simulink model "Control_Jetson_10ms_21b 1"  (R2021b)
settings: Solver=ode4  StartTime=0.0  StopTime=10  FixedStep=0.01  MaxStep=0  RelTol=1e-5  AbsTol=1e-3
InitFcn:
  | % Carrega parâmetros gerais (Massa, Ganhos PID, Geometria)
  | run('Parameters.m');
  | 
  | % Carrega as Tabelas (Lookup Tables)
  | run('curva_steering.m');
  | run('curva_tq_motor.m');
  | Ts = 0.001;
  | % (Opcional) Mensagem no Command Window para confirmar que rodou
  | disp('--- Parâmetros e Curvas Carregados com Sucesso ---');
model workspace (MAT data in the model file):
  A = 1.22
  Ack = 1
  Cd = 1.1
  Cl = -2
  Cs = [19075.58 25992.8 31792.64 35898.02 39044.37]
  Fz0x = -811.9083
  Fz0y = -210.9467
  Fz_cs = [222.41 444.82 667.23 889.64 1112.05]
  IAY = 0
  IAx = 0
  IAy = 0
  Im = 0.00033
  It = 0.0094
  Iw = 0.1578
  Iw_ = 0.7
  Iz_car = 150
  K_50_understeer = 0.005184
  K_Stability = 1
  K_oversteer = -0.001
  Kappa_F = 0
  Kappa_R = 0
  Km_FM = 110000
  Km_Fm = 110000
  Km_RM = 120000
  Km_Rm = 120000
  KphiARB_F = 0
  KphiARB_R = 11000
  KphiF = 1068.14
  KphiR = 1637.12
  Kphim_F = 137500
  Kphim_R = 48600
  L = 1.53
  M = 300
  Mgt = 11.72
  Mz_maxF = [0 66.3 132.6 198.9 265.2 330.23 396.52 462.83 529.112 595.42 661.73 728.03 794.33 860.62 926.92 993.23 1058.25 1124.55 1190.85 1257.15 1323.45 1389.75 1456.05 1522.35 1588.65 1654.95]
  Mz_minF = [0 -66.3 -132.6 -198.9 -265.2 -330.23 -396.52 -462.83 -529.112 -595.42 -661.73 -728.03 -794.33 -860.62 -926.92 -993.23 -1058.25 -1124.55 -1190.85 -1257.15 -1323.45 -1389.75 -1456.05 -1522.35 -1588.65 -1654.95]
  P = 68.9476
  P0 = 55.4852
  R = 0.2032
  Rcurva = 20
  Re = 0.2
  SR = 3
  TV_On = 1
  Ts = 0.01
  W = 2940
  Wf = 661.5
  Wr = 808.5
  Ws = 2324
  YLL = 1.11022302463e-16
  cx1 = 1.3668
  cy1 = 1.839
  dpi = 0.242630467224
  dx1 = 2.1568
  dx2 = -0.065814
  dx3 = 0.0011254
  dy1 = 2.453
  dy2 = -0.11197
  dy3 = 10.2899
  ex1 = -0.19815
  ex2 = -0.62529
  ex3 = 1.3396
  ex4 = 0.0029464
  ey1 = 0.96085
  ey2 = -0.28662
  ey3 = 0.14389
  ey4 = 4.9274
  ey5 = -70.7165
  g = 9.8
  hcg = 0.28495
  hcgs = 0.202
  hrc_f = 0.065
  hrc_r = 0.094
  hs_f = 0.245
  hs_r = 0.21
  hx1 = -0.003859
  hx2 = -0.000374
  hy1 = -0.000403
  hy2 = -0.000261
  kx1 = -36.9039
  kx2 = 22.3857
  kx3 = 0.61844
  ky1 = -83.2526
  ky2 = -5.565
  ky3 = 0.88491
  ky4 = 2.9994
  ky5 = -99.9393
  ky6 = -3.4705
  ky7 = -0.91452
  lf = 0.8415
  lr = 0.6885
  mass_FL = 67.5
  mass_FR = 67.5
  mass_RL = 82.5
  mass_RR = 82.5
  mi = 2
  ms = 240
  pedal = [0 1 2 3 4 5 6 7 8 9 10 11 12 13 14 15 16 17 18 19 20 21 22 23 24 25]
  pty1 = 0.005744
  pty2 = 19.1334
  px1 = -0.039964
  px2 = -0.15015
  px3 = -0.32528
  px4 = -0.063273
  py1 = 0.38578
  py2 = 1.2048
  py3 = -0.14544
  py4 = 0.092886
  py5 = -0.82901
  r = 9
  rhoar = 1.22
  s_f = 1
  s_r = 0.9
  tf = 1.2
  tr = 1.18
  vx1 = -0.11922
  vx2 = 0.002205
  vy1 = 0.032907
  vy2 = 0.018068
  vy3 = -1.0429
  vy4 = 0.53712
  x_fl = 0.8415
  x_fr = 0.8415
  x_rl = 0.6885
  x_rr = 0.6885
  xs_f = 0.89
  xs_r = 0.638
  y_fl = 0.6
  y_fr = 0.6
  y_rl = 0.59
  y_rr = 0.59
undefined symbols (not defined in the file or in its folder): Gr, K_t, K_variavel, Ki_data, Kp_data, magnitude, rpm, torque, Vx, Vx_axis
libraries: simulink x10, fuzblock x4
(part 1 of 2)
settings Model: SimulationMode=accelerator  NumberOfSteps=275  Creator=lucas  LastModifiedBy=Aline
settings SolverCC: ZeroCrossAlgorithm=Adaptive
settings DebuggingCC: SignalInfNanChecking=error  IgnoredZcDiagnostic=none  UnconnectedInputMsg=none  UnconnectedOutputMsg=none  UnconnectedLineMsg=none
settings ModelReferenceCC: EnableRefExpFcnMdlSchedulingChecks=off
settings RTWCC: GPUComputeCapability=5.0  DLArmComputeVersion=20.02.1

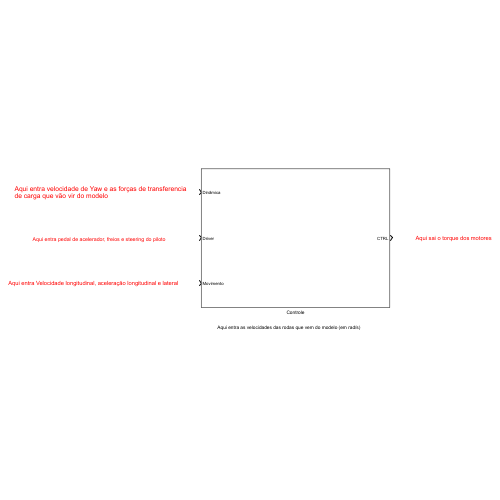
[thumbnail: Simulink's stored preview of the top-level diagram]
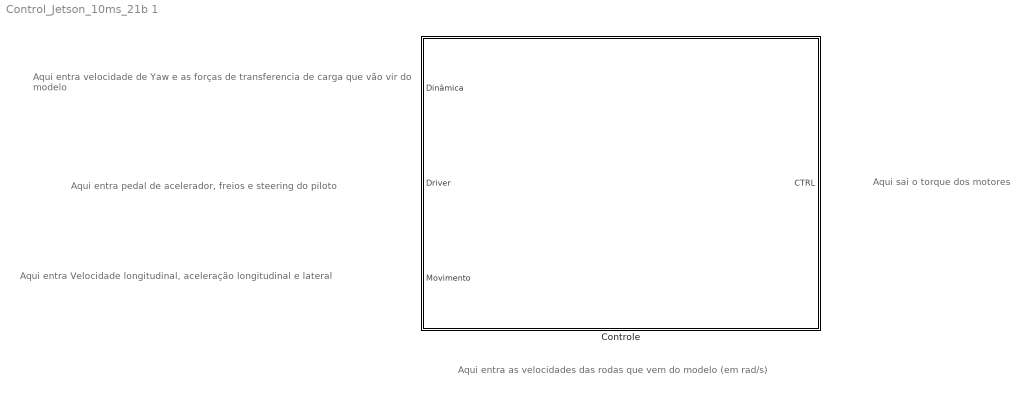
== system Control_Jetson_10ms_21b 1 ==
  note: Aqui sai o torque dos motores
  note: Aqui entra as velocidades das rodas que vem do modelo (em rad/s)
  note: Aqui entra Velocidade longitudinal, aceleração longitudinal e lateral
  note: Aqui entra pedal de acelerador, freios e steering do piloto
  note: Aqui entra velocidade de Yaw e as forças de transferencia
      | de carga que vão vir do modelo
  Controle : Subsystem

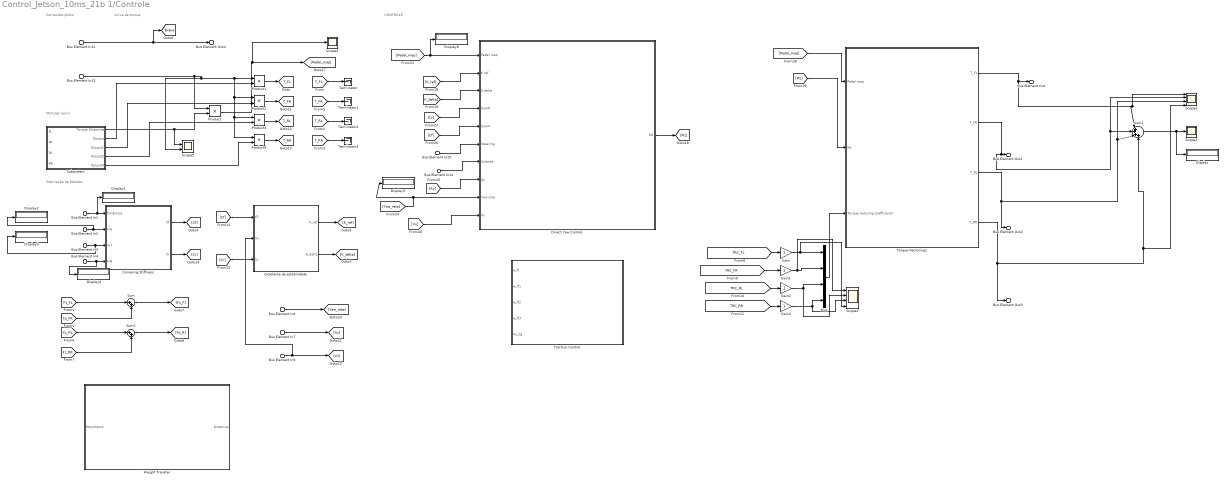
== system Control_Jetson_10ms_21b 1/Controle ==
  note: CONTROLE
  note: Estimação de Estados
  note: Motores
      |  (rpm)
  note: Comandos piloto
  note: curva de torque
  Bus Element In1 : Inport  PortName=Dinâmica  Element=Fz_FL
  Bus Element In2 : Inport  PortName=Dinâmica  Element=Fz_FR
  Bus Element In3 : Inport  PortName=Dinâmica  Element=Fz_RL
  Bus Element In4 : Inport  PortName=Dinâmica  Element=Fz_RR
  Bus Element In6 : Inport  PortName=Dinâmica  Element=Yaw.v_yaw
  Bus Element In12 : Inport  Port=2  PortName=Driver  Element=BrakeCmd
  Bus Element In13 : Inport  Port=2  PortName=Driver  Element=AccCmd
  Bus Element In14 : Inport  Port=2  PortName=Driver  Element=volante
  Bus Element In15 : Inport  Port=2  PortName=Driver  Element=steering_inner
  Bus Element In5 : Inport  Port=3  PortName=Movimento  Element=Vx_cg
  Bus Element In7 : Inport  Port=3  PortName=Movimento  Element=Ay_cg
  Cornering Stiffness : Subsystem
  Direct Yaw Control : Subsystem
  Display{,1..6} (7 alike) : Display
  Gain{,1..3} (4 alike) : Gain
  Gradiente de estabilidade : Subsystem
  Mux : Mux
  Product{,1..4} (5 alike) : Product
  Scope1 : Scope
  Scope2 : Scope  NumInputPorts=4
  Scope3 : Scope  NumInputPorts=4
  Scope4 : Scope
  Scope5 : Scope  NumInputPorts=2
  Subsystem : Subsystem
  Sum : Sum  Inputs=|++
  Sum1 : Sum  Inputs=|++
  Sum2 : Sum  Inputs=|++++
  Terminator{,1..3} (4 alike) : Terminator
  Torque Vectoring1 : Subsystem
  Traction Control : Subsystem
  "Weight Transfer " : Subsystem
  Bus Element Out4 : Outport  PortName=CTRL  Element=BrakeCmd
  Bus Element Out : Outport  VectorParamsAs1DForOutWhenUnconnected=off  PortName=CTRL  Element=T_FL
  Bus Element Out1 : Outport  VectorParamsAs1DForOutWhenUnconnected=off  PortName=CTRL  Element=T_FR
  Bus Element Out2 : Outport  VectorParamsAs1DForOutWhenUnconnected=off  PortName=CTRL  Element=T_RL
  Bus Element Out3 : Outport  VectorParamsAs1DForOutWhenUnconnected=off  PortName=CTRL  Element=T_RR
  tag scope: Brake=global, T_FL=global, T_FR=global, T_RL=global, T_RR=global
  wires:
  Gradiente de estabilidade/2(K_delta) -> [K_delta]
  Bus Element In13/1 -> Scope5/2, Product4/1, Product3/1, Product2/1, Product1/1, Product/1
  Bus Element In12/1 -> [Brake], Bus Element Out4/1
  Cornering Stiffness/1(Cf) -> [Cf]
  Cornering Stiffness/2(Cr) -> [Cr]
  Bus Element In3/1 -> Display3/1, Cornering Stiffness/3(In7)
  Bus Element In1/1 -> Display1/1, Cornering Stiffness/1(Dinâmica)
  Bus Element In4/1 -> Display4/1, Cornering Stiffness/4(In8)
  Bus Element In2/1 -> Display2/1, Cornering Stiffness/2(In6)
  [Cr] -> Gradiente de estabilidade/3(Cr)
  [Cf] -> Gradiente de estabilidade/1(Cf)
  Gradiente de estabilidade/1(K_ref) -> [K_ref]
  Direct Yaw Control/1(Mz) -> [Mz]
  Bus Element In14/1 -> Direct Yaw Control/7(Volante)
  Bus Element In15/1 -> Direct Yaw Control/6(Steering)
  [Mz] -> Torque Vectoring1/2(Mz)
  Sum/1 -> [Fz_F]
  Sum1/1 -> [Fz_R]
  Bus Element In5/1 -> Gradiente de estabilidade/2(Vx), [Vx]
  Bus Element In7/1 -> [Ay]
  Bus Element In6/1 -> [Yaw_rate]
  [T_FL] -> Terminator/1
  [T_FR] -> Terminator1/1
  [T_RL] -> Terminator2/1
  [T_RR] -> Terminator3/1
  Sum2/1 -> Display/1, Scope1/1
  Mux/1 -> Torque Vectoring1/3(Torque reducing coefficients)
  Product/1 -> [Pedal_map], Scope4/1
  Subsystem/1(Torque Disponivel) -> Product/2, Scope5/1
  Product1/1 -> [T_FL]
  Product2/1 -> [T_FR]
  Product3/1 -> [T_RL]
  Product4/1 -> [T_RR]
  Subsystem/5(Output3) -> Product4/2
  Subsystem/4(Output2) -> Product3/2
  Subsystem/3(Output1) -> Product2/2
  Subsystem/2(Output) -> Product1/2
  ? -> Subsystem/3(RL)
  ? -> Subsystem/4(RR)
  ? -> Subsystem/2(FR)
  ? -> Subsystem/1(FL)
  Torque Vectoring1/2(T_FR) -> Scope3/2, Sum2/2, Bus Element Out1/1
  Torque Vectoring1/3(T_RL) -> Bus Element Out2/1, Scope3/3, Sum2/3
  Torque Vectoring1/1(T_FL) -> Sum2/1, Scope3/1, Bus Element Out/1
  Torque Vectoring1/4(T_RR) -> Bus Element Out3/1, Scope3/4, Sum2/4
  [TRC_FL] -> Gain/1
  [TRC_FR] -> Gain1/1
  Gain/1 -> Scope2/4, Mux/1
  Gain1/1 -> Scope2/1, Mux/2
  [TRC_RL] -> Gain2/1
  [TRC_RR] -> Gain3/1
  [Pedal_map] -> Direct Yaw Control/1(Pedal map), Display6/1
  [K_ref] -> Direct Yaw Control/2(K ref)
  [K_delta] -> Direct Yaw Control/3(K delta)
  [Cr] -> Direct Yaw Control/4(CornR)
  [Cf] -> Direct Yaw Control/5(CornF)
  [Ay] -> Direct Yaw Control/8(Ay)
  [Vx] -> Direct Yaw Control/10(Vx)
  [Pedal_map] -> Torque Vectoring1/1(Pedal map)
  Gain2/1 -> Mux/3, Scope2/2
  Gain3/1 -> Mux/4, Scope2/3
  [Yaw_rate] -> Direct Yaw Control/9(Yaw rate), Display5/1
  [Fz_FR] -> Sum/2
  [Fz_FL] -> Sum/1
  [Fz_RR] -> Sum1/2
  [Fz_RL] -> Sum1/1

== system Control_Jetson_10ms_21b 1/Controle/Cornering Stiffness ==
  Dinâmica : Inport
  In6 : Inport  Port=2
  In7 : Inport  Port=3
  In8 : Inport  Port=4
  1-D Lookup Table{,1..3} (4 alike) : Lookup_n-D  NumberOfTableDimensions=1  BreakpointsForDimension1=Fz_cs  Table=Cs  InternalRulePriority=Speed  RndMeth=Simplest  InputSameDT=on
  Sum : Sum  Inputs=|++
  Sum1 : Sum  Inputs=|++
  Cf : Outport
  Cr : Outport  Port=2
  wires:
  1-D Lookup Table1/1 -> Sum1/2
  In7/1 -> 1-D Lookup Table2/1
  Sum/1 -> Cr/1
  Sum1/1 -> Cf/1
  Dinâmica/1 -> 1-D Lookup Table/1
  In6/1 -> 1-D Lookup Table1/1
  1-D Lookup Table3/1 -> Sum/2
  1-D Lookup Table/1 -> Sum1/1
  1-D Lookup Table2/1 -> Sum/1
  In8/1 -> 1-D Lookup Table3/1

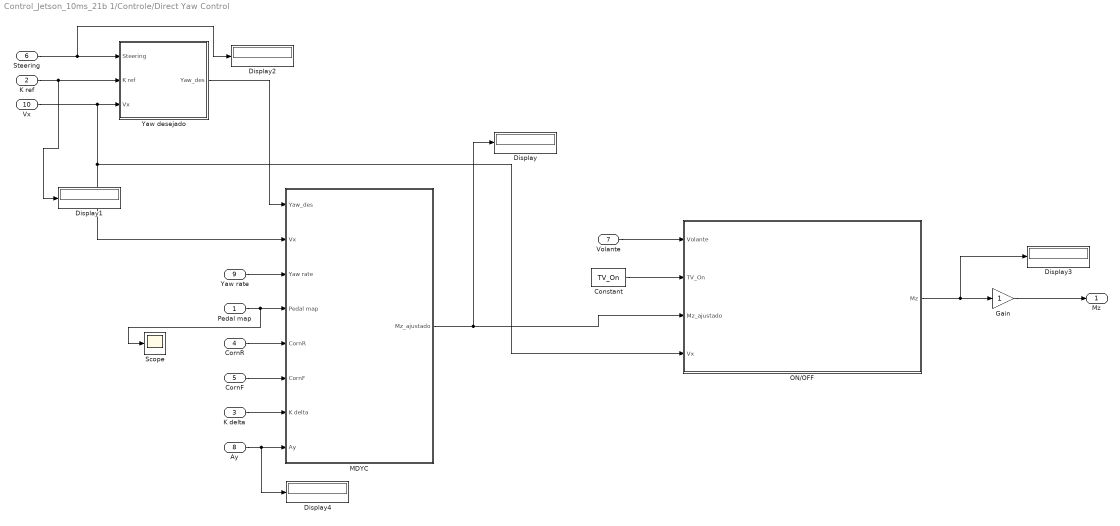
== system Control_Jetson_10ms_21b 1/Controle/Direct Yaw Control ==
  Pedal map : Inport
  K ref : Inport  Port=2
  K delta : Inport  Port=3
  CornR : Inport  Port=4
  CornF : Inport  Port=5
  Steering : Inport  Port=6
  Volante : Inport  Port=7
  Ay : Inport  Port=8
  Yaw rate : Inport  Port=9
  Vx : Inport  Port=10
  Constant : Constant  Value=TV_On
  Display{,1..4} (5 alike) : Display
  Gain : Gain
  MDYC : Subsystem
  ON/OFF : Subsystem
  Scope : Scope
  Yaw desejado : Subsystem
  Mz : Outport
  wires:
  Steering/1 -> Display2/1, Yaw desejado/1(Steering)
  K ref/1 -> Display1/1, Yaw desejado/2(K ref)
  Vx/1 -> MDYC/2(Vx), ON/OFF/4(Vx), Yaw desejado/3(Vx)
  Yaw desejado/1(Yaw_des) -> MDYC/1(Yaw_des)
  Yaw rate/1 -> MDYC/3(Yaw rate)
  Pedal map/1 -> Scope/1, MDYC/4(Pedal map)
  CornR/1 -> MDYC/5(CornR)
  CornF/1 -> MDYC/6(CornF)
  K delta/1 -> MDYC/7(K delta)
  Ay/1 -> Display4/1, MDYC/8(Ay)
  Volante/1 -> ON/OFF/1(Volante)
  Constant/1 -> ON/OFF/2(TV_On)
  MDYC/1(Mz_ajustado) -> Display/1, ON/OFF/3(Mz_ajustado)
  ON/OFF/1(Mz) -> Display3/1, Gain/1
  Gain/1 -> Mz/1

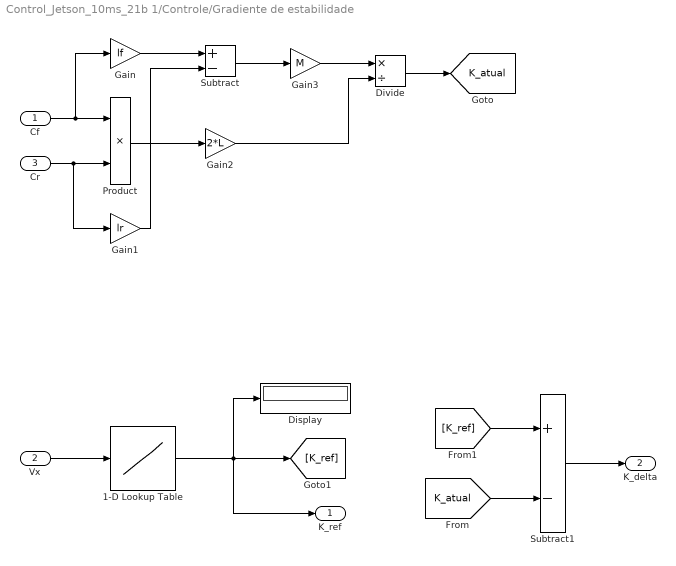
== system Control_Jetson_10ms_21b 1/Controle/Gradiente de estabilidade ==
  Cf : Inport
  Vx : Inport  Port=2
  Cr : Inport  Port=3
  1-D Lookup Table : Lookup_n-D  NumberOfTableDimensions=1  BreakpointsForDimension1=Vx  Table=K_variavel  InternalRulePriority=Speed  RndMeth=Simplest  InputSameDT=on
  Display : Display
  Divide : Product  Inputs=*/
  Gain : Gain  Gain=lf
  Gain1 : Gain  Gain=lr
  Gain2 : Gain  Gain=2*L
  Gain3 : Gain  Gain=M
  Product : Product
  Subtract : Sum  Inputs=+-
  Subtract1 : Sum  Inputs=+-
  K_ref : Outport
  K_delta : Outport  Port=2
  tag scope: K_atual=global
  wires:
  Cr/1 -> Product/2, Gain1/1
  [K_ref] -> Subtract1/1
  Product/1 -> Gain2/1
  Divide/1 -> [K_atual]
  Subtract1/1 -> K_delta/1
  Gain2/1 -> Divide/2
  [K_atual] -> Subtract1/2
  Gain3/1 -> Divide/1
  Cf/1 -> Gain/1, Product/1
  Gain1/1 -> Subtract/2
  Gain/1 -> Subtract/1
  Subtract/1 -> Gain3/1
  Vx/1 -> 1-D Lookup Table/1
  1-D Lookup Table/1 -> Display/1, K_ref/1, [K_ref]

== system Control_Jetson_10ms_21b 1/Controle/Subsystem ==
  Bus Element In1 : Inport  PortName=FL
  Bus Element In2 : Inport  Port=2  PortName=FR
  Bus Element In3 : Inport  Port=3  PortName=RL
  Bus Element In4 : Inport  Port=4  PortName=RR
  1-D Lookup Table{,1..3} (4 alike) : Lookup_n-D  NumberOfTableDimensions=1  BreakpointsForDimension1=rpm  Table=torque  InternalRulePriority=Speed  RndMeth=Simplest  InputSameDT=on
  Sum : Sum  Inputs=|++++
  Torque Disponivel : Outport
  Output : Outport  Port=2
  Output1 : Outport  Port=3
  Output2 : Outport  Port=4
  Output3 : Outport  Port=5
  wires:
  1-D Lookup Table/1 -> Output/1, Output1/1, Sum/1
  1-D Lookup Table1/1 -> Sum/2
  1-D Lookup Table2/1 -> Output2/1, Sum/3
  1-D Lookup Table3/1 -> Output3/1, Sum/4
  Sum/1 -> Torque Disponivel/1
  Bus Element In1/1 -> 1-D Lookup Table/1
  Bus Element In2/1 -> 1-D Lookup Table1/1
  Bus Element In3/1 -> 1-D Lookup Table2/1
  Bus Element In4/1 -> 1-D Lookup Table3/1

== system Control_Jetson_10ms_21b 1/Controle/Torque Vectoring1 ==
  note: rever isso daqui
  Pedal map : Inport
  Mz : Inport  Port=2
  Torque reducing coefficients : Inport  Port=3
  Display : Display
  Display1 : Display
  Distribuição Lateral2 : Subsystem
  Distribuição longitudinal : Subsystem
  Redução TC1 : Subsystem
  Scope : Scope  NumInputPorts=4
  Scope1 : Scope  NumInputPorts=2
  Subsystem : Subsystem
  T_FL : Outport
  T_FR : Outport  Port=2
  T_RL : Outport  Port=3
  T_RR : Outport  Port=4
  tag scope: Tq_F=global, Tq_R=global
  wires:
  Redução TC1/3(T_RLreduzido) -> Scope/3, T_RL/1  "RL"
  Torque reducing coefficients/1 -> Redução TC1/1(Torque reducing coefficients)
  Subsystem/2("Tq_R ") -> Distribuição Lateral2/4("Tq_R "), [Tq_R]
  Mz/1 -> Subsystem/1(MzT)
  Redução TC1/2(T_FRreduzido) -> Scope/2, T_FR/1  "FR"
  Redução TC1/1(T_FLreduzido) -> Scope1/2, Scope/1, T_FL/1  "FL"
  Subsystem/1(Tq_F) -> Distribuição Lateral2/3(Tq_F), [Tq_F]
  Redução TC1/4(T_RRreduzido) -> Scope/4, T_RR/1  "RR"
  Distribuição longitudinal/1(Dianteiro) -> Distribuição Lateral2/1(Dianteiro)
  Distribuição longitudinal/2(Traseiro) -> Distribuição Lateral2/2(Traseiro)
  Pedal map/1 -> Distribuição longitudinal/1(In1)
  Distribuição Lateral2/1(TFL_lat) -> Redução TC1/2(TFL)
  Distribuição Lateral2/2(TFR_lat) -> Redução TC1/3(TFR)
  Distribuição Lateral2/3(TRL_lat) -> Redução TC1/4(TRL)
  Distribuição Lateral2/4(TRR_lat) -> Redução TC1/5(TRR)

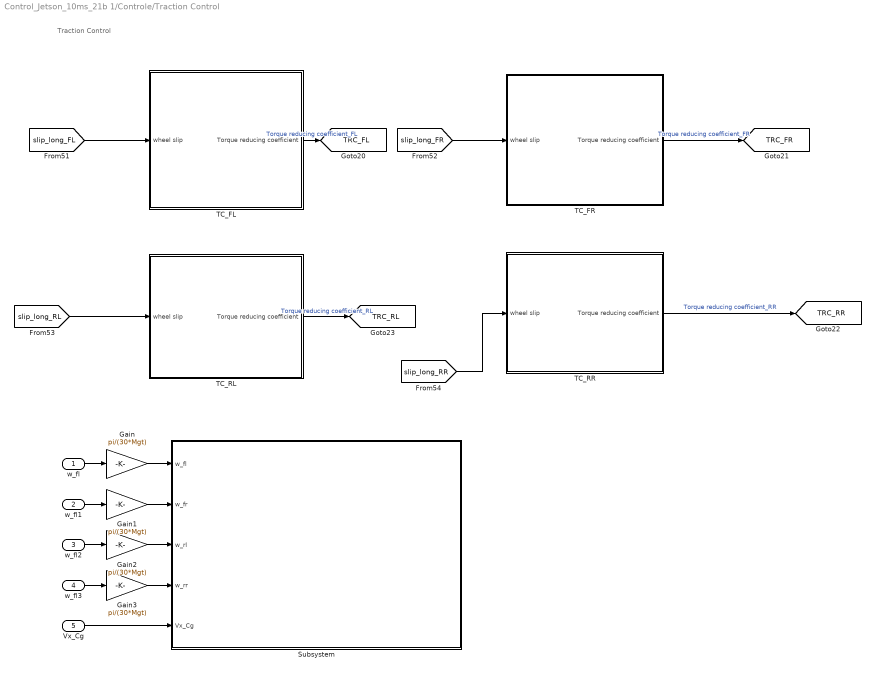
== system Control_Jetson_10ms_21b 1/Controle/Traction Control ==
  note: Traction Control
  w_fl : Inport
  w_fl1 : Inport  Port=2
  w_fl2 : Inport  Port=3
  w_fl3 : Inport  Port=4
  Vx_Cg : Inport  Port=5
  Gain{,1..3} (4 alike) : Gain  Gain=pi/(30*Mgt)
  Subsystem : Subsystem
  TC_FL : Subsystem
  TC_FR : Subsystem
  TC_RL : Subsystem
  TC_RR : Subsystem
  tag scope: TRC_FL=global, TRC_FR=global, TRC_RL=global, TRC_RR=global
  wires:
  TC_FR/1(Torque reducing coefficient) -> [TRC_FR]  "Torque reducing coefficient_FR"
  TC_RL/1(Torque reducing coefficient) -> [TRC_RL]  "Torque reducing coefficient_RL"
  TC_FL/1(Torque reducing coefficient) -> [TRC_FL]  "Torque reducing coefficient_FL"
  [slip_long_FL] -> TC_FL/1(wheel slip)
  [slip_long_RL] -> TC_RL/1(wheel slip)
  [slip_long_RR] -> TC_RR/1(wheel slip)
  [slip_long_FR] -> TC_FR/1(wheel slip)
  TC_RR/1(Torque reducing coefficient) -> [TRC_RR]  "Torque reducing coefficient_RR"
  w_fl/1 -> Gain/1
  w_fl1/1 -> Gain1/1
  w_fl2/1 -> Gain2/1
  w_fl3/1 -> Gain3/1
  Gain/1 -> Subsystem/1(w_fl)
  Gain1/1 -> Subsystem/2(w_fr)
  Gain2/1 -> Subsystem/3(w_rl)
  Gain3/1 -> Subsystem/4(w_rr)
  Vx_Cg/1 -> Subsystem/5(Vx_Cg)

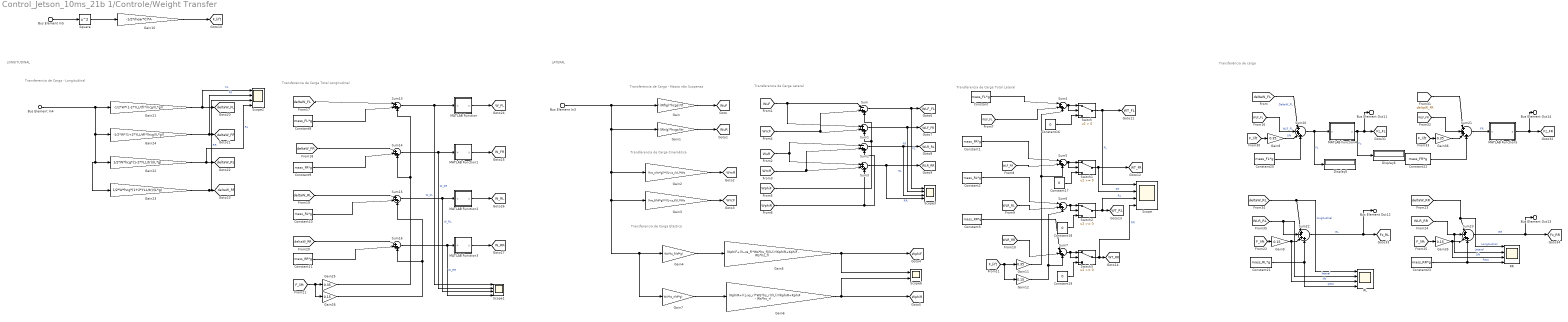
== system Control_Jetson_10ms_21b 1/Controle/Weight Transfer  ==
  note: Transferencia de Carga Lateral
  note: LATERAL
  note: Transferencia de Carga Cinemática
  note: Transferência de carga
  note: Transferencia de Carga - Massa não Suspensa
  note: Transferencia de Carga Total Lateral
  note: LONGITUDINAL
  note: Transferencia de Carga - Longitudinal
  note: Transferencia de Carga Total Longitudinal
  note: Transferencia de Carga Elástica
  Bus Element In3 : Inport  PortName=Movimento  Element=Ay_cg
  Bus Element In4 : Inport  PortName=Movimento  Element=Ax_cg
  Bus Element In5 : Inport  PortName=Movimento  Element=Vx_cg
  Constant : Constant  Value=mass_FL*g
  Constant1 : Constant  Value=mass_FR*g
  Constant10 : Constant  Value=mass_RL*g
  Constant11 : Constant  Value=mass_RR*g
  Constant{16..19} (4 alike) : Constant  Value=0
  Constant2 : Constant  Value=mass_RL*g
  Constant20 : Constant  Value=mass_FL*g
  Constant21 : Constant  Value=mass_RL*g
  Constant22 : Constant  Value=mass_FR*g
  Constant23 : Constant  Value=mass_RR*g
  Constant3 : Constant  Value=mass_RR*g
  Constant8 : Constant  Value=mass_FL*g
  Constant9 : Constant  Value=mass_FR*g
  Display5 : Display
  Display6 : Display
  Gain : Gain  Gain=((Wf/g)*hcgs)/tf
  Gain1 : Gain  Gain=((Wr/g)*hcgs)/tr
  Gain10 : Gain  Gain=-1/2*rhoar*Cl*A
  Gain{8,11,25,36} (4 alike) : Gain  Gain=0.35
  Gain{9,12,26,35} (4 alike) : Gain  Gain=0.15
  Gain2 : Gain  Gain=(hrc_r/(tr*g))*((L-xs_r)/L)*Ws
  Gain21 : Gain  Gain=-1/2*W*(1-2*YLL/tf)*(hcg/(L*g))
  Gain22 : Gain  Gain=1/2*W*hcg*(1-2*YLL/tr)/(L*g)
  Gain23 : Gain  Gain=1/2*W*hcg*(1+2*YLL/tr)/(L*g)
  Gain24 : Gain  Gain=-1/2*W*(1+2*YLL/tf)*(hcg/(L*g))
  Gain3 : Gain  Gain=(hrc_f/(tf*g))*((L-xs_f)/L)*Ws
  Gain4 : Gain  Gain=Ws*hs_f/(tf*g)
  Gain5 : Gain  Gain=(KphiF+((L-xs_f)*Ws*hs_f)/(L))/(KphiR+KphiF - Ws*hs_f)
  Gain6 : Gain  Gain=(KphiR+((L-xs_r)*Ws*hs_r)/(L))/(KphiR+KphiF - Ws*hs_r)
  Gain7 : Gain  Gain=Ws*hs_r/(tf*g)
  MATLAB Function : MATLAB Function  TreatAsAtomicUnit=on
  MATLAB Function1 : MATLAB Function  TreatAsAtomicUnit=on
  MATLAB Function2 : MATLAB Function  TreatAsAtomicUnit=on
  MATLAB Function3 : MATLAB Function  TreatAsAtomicUnit=on
  MATLAB Function4 : MATLAB Function  TreatAsAtomicUnit=on
  MATLAB Function5 : MATLAB Function  TreatAsAtomicUnit=on
  RL : Scope  NumInputPorts=4
  RR : Scope  NumInputPorts=4
  Scope{,1..3} (4 alike) : Scope  NumInputPorts=4
  Scope6 : Scope  NumInputPorts=2
  Square : Math  Operator=square  SaturateOnIntegerOverflow=on
  Sum : Sum  Inputs=|-++
  Sum{1,3..7,13..16} (10 alike) : Sum  Inputs=|+++
  Sum2 : Sum  Inputs=|-++
  Sum{20..23} (4 alike) : Sum  Inputs=|++++
  Switch : Switch  Criteria=u2 > Threshold
  Switch1 : Switch
  Switch2 : Switch
  Switch3 : Switch
  Bus Element Out11 : Outport  VectorParamsAs1DForOutWhenUnconnected=off  PortName=Dinâmica  Element=Fz_FL
  Bus Element Out12 : Outport  VectorParamsAs1DForOutWhenUnconnected=off  PortName=Dinâmica  Element=Fz_RL
  Bus Element Out13 : Outport  VectorParamsAs1DForOutWhenUnconnected=off  PortName=Dinâmica  Element=Fz_RR
  Bus Element Out14 : Outport  VectorParamsAs1DForOutWhenUnconnected=off  PortName=Dinâmica  Element=Fz_FR
  tag scope: F_lift=global, Fz_FL=global, Fz_FR=global, Fz_RL=global, Fz_RR=global, WLF_FL=global, WLF_FR=global, WLR_RL=global, WLR_RR=global, WT_FL=global, WT_FR=global, WT_RL=global, WT_RR=global, W_FL=global, W_FR=global, W_RL=global, W_RR=global, WphiF=global, WphiR=global, WrcF=global, WrcR=global, WuF=global, WuR=global, deltaW_FL=global, deltaW_FR=global, deltaW_RL=global, deltaW_RR=global
  wires:
  Sum22/1 -> Bus Element Out12/1, [Fz_RL]  "RL"
  Constant10/1 -> Sum15/2
  Gain25/1 -> Sum14/3, Sum13/3
  Sum23/1 -> [Fz_RR], Bus Element Out13/1  "RR"
  [F_lift] -> Gain35/1
  Constant22/1 -> Sum21/4
  [WLF_FR] -> Sum5/2
  Switch1/1 -> Scope/2, [WT_FR]  "FR"
  Gain10/1 -> [F_lift]
  [F_lift] -> Gain36/1
  [WrcF] -> Sum1/2, Sum/2
  [deltaW_FL] -> Sum13/1
  [WLR_RR] -> RR/2, Sum23/2  "Lateral"
  Sum1/1 -> [WLF_FR], Scope3/2  "FR"
  Bus Element In4/1 -> Gain24/1, Gain23/1, Gain22/1, Gain21/1
  Gain12/1 -> Sum7/3, Sum6/3
  Switch2/1 -> Scope/3, [WT_RL]  "RL"
  MATLAB Function3/1(y) -> [W_RR]
  Constant17/1 -> Switch1/3
  Switch3/1 -> Scope/4, [WT_RR]  "RR"
  MATLAB Function1/1(y) -> [W_FR]
  Sum3/1 -> [WLR_RR], Scope3/4  "RR"
  Constant21/1 -> Sum22/4, RL/4  "peso"
  MATLAB Function2/1(y) -> [W_RL]
  [WrcR] -> Sum2/2, Sum3/2
  [deltaW_RL] -> Sum22/1, RL/1  "longitudinal"
  [WphiF] -> Sum/3, Sum1/3
  Constant3/1 -> Sum7/1
  [WLF_FR] -> Sum21/2
  [F_lift] -> Gain9/1
  Sum16/1 -> Scope1/4, MATLAB Function3/1(u)  "W_RR"
  Sum2/1 -> [WLR_RL], Scope3/3  "RL"
  Sum4/1 -> Switch/2, Switch/1
  MATLAB Function4/1(y) -> Display6/1, Bus Element Out11/1, [Fz_FL]  "Fz"
  Gain7/1 -> Gain6/1
  Gain23/1 -> Scope2/3, [deltaW_RR]  "RR"
  Constant8/1 -> Sum13/2
  [WLR_RL] -> Sum22/2, RL/2  "lateral"
  Constant23/1 -> RR/4, Sum23/4  "Peso"
  Gain22/1 -> Scope2/4, [deltaW_RL]  "RL"
  [deltaW_RL] -> Sum15/1
  Gain26/1 -> Sum16/3, Sum15/3
  [F_lift] -> Gain8/1
  Constant20/1 -> Sum20/4
  Bus Element In3/1 -> Gain/1, Gain7/1, Gain4/1, Gain3/1, Gain2/1, Gain1/1
  Sum15/1 -> Scope1/3, MATLAB Function2/1(u)  "W_RL"
  Constant11/1 -> Sum16/2
  Gain8/1 -> Sum20/3  "Lift"
  Gain21/1 -> Scope2/1, [deltaW_FL]  "FL"
  MATLAB Function5/1(y) -> Bus Element Out14/1, [Fz_FR]
  Constant9/1 -> Sum14/2
  Gain5/1 -> [WphiF], Scope6/1
  Switch/1 -> Scope/1, [WT_FL]  "FL"
  [F_lift] -> Gain12/1, Gain11/1
  Gain3/1 -> [WrcF]
  Sum7/1 -> Switch3/2, Switch3/1
  [deltaW_FR] -> Sum14/1
  [deltaW_FR] -> Sum21/1
  Sum20/1 -> Display5/1, MATLAB Function4/1(u)  "FL"
  Sum6/1 -> Switch2/2, Switch2/1
  Square/1 -> Gain10/1
  [WLF_FL] -> Sum20/2  "WLF_FL"
  [WuR] -> Sum2/1, Sum3/1
  Gain1/1 -> [WuR]
  Gain4/1 -> Gain5/1
  [deltaW_RR] -> RR/1, Sum23/1  "Longitudinal"
  Gain/1 -> [WuF]
  [WphiR] -> Sum3/3, Sum2/3
  [WLR_RL] -> Sum6/2
  [WuF] -> Sum1/1, Sum/1
  Bus Element In5/1 -> Square/1
  Gain2/1 -> [WrcR]
  Constant18/1 -> Switch2/3
  Gain24/1 -> Scope2/2, [deltaW_FR]  "FR"
  Sum5/1 -> Switch1/2, Switch1/1
  [WLR_RR] -> Sum7/2
  Sum14/1 -> Scope1/2, MATLAB Function1/1(u)  "W_FR"
  [F_lift] -> Gain26/1, Gain25/1
  Gain36/1 -> Sum21/3
  [deltaW_FL] -> Sum20/1  "DeltaW_FL"
  MATLAB Function/1(y) -> [W_FL]
  Sum/1 -> [WLF_FL], Scope3/1  "FL"
  Constant19/1 -> Switch3/3
  Constant16/1 -> Switch/3
  [deltaW_RR] -> Sum16/1
  Sum21/1 -> MATLAB Function5/1(u)  "FR"
  Sum13/1 -> MATLAB Function/1(u), Scope1/1  "W_FL"
  Gain11/1 -> Sum5/3, Sum4/3
  Gain9/1 -> RL/3, Sum22/3  "lift"
  [WLF_FL] -> Sum4/2
  Constant1/1 -> Sum5/1
  Constant2/1 -> Sum6/1
  Gain35/1 -> RR/3, Sum23/3  "Lift"
  Gain6/1 -> Scope6/2, [WphiR]
  Constant/1 -> Sum4/1

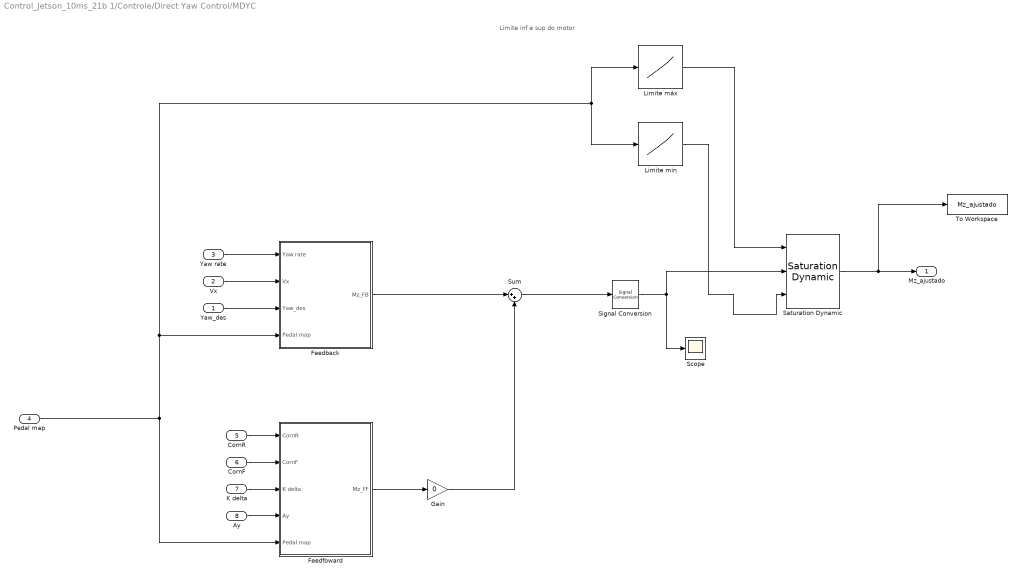
== system Control_Jetson_10ms_21b 1/Controle/Direct Yaw Control/MDYC ==
  note: Limite inf e sup do motor
  Yaw_des : Inport
  Vx : Inport  Port=2
  Yaw rate : Inport  Port=3
  Pedal map : Inport  Port=4
  CornR : Inport  Port=5
  CornF : Inport  Port=6
  K delta : Inport  Port=7
  Ay : Inport  Port=8
  Feedback : Subsystem
  Feedfoward : Subsystem
  Gain : Gain  Gain=0
  Limite min : Lookup_n-D  NumberOfTableDimensions=1  BreakpointsForDimension1=pedal  BreakpointsForDimension3=[5, 7]  Table=Mz_minF  InternalRulePriority=Speed  RndMeth=Simplest  InputSameDT=on
  Limite máx : Lookup_n-D  NumberOfTableDimensions=1  BreakpointsForDimension1=pedal  BreakpointsForDimension3=[5, 7]  Table=Mz_maxF  InternalRulePriority=Speed  RndMeth=Simplest  InputSameDT=on
  Saturation Dynamic : simulink/Discontinuities/Saturation Dynamic  OutMin=[]  OutMax=[]  OutDataTypeStr=Inherit: Same as second input  OutDataType=fixdt(1, 16)  OutScaling=2^-10  DoSatur=off
  Scope : Scope
  Signal Conversion : SignalConversion  OverrideOpt=off
  Sum : Sum  Inputs=|++
  To Workspace : ToWorkspace  VariableName=Mz_ajustado  SaveFormat=Structure With Time  SampleTime=-1
  Mz_ajustado : Outport
  wires:
  K delta/1 -> Feedfoward/3(K delta)
  Feedback/1(Mz_FB) -> Sum/1
  Ay/1 -> Feedfoward/4(Ay)
  CornR/1 -> Feedfoward/1(CornR)
  Yaw rate/1 -> Feedback/1(Yaw rate)
  Vx/1 -> Feedback/2(Vx)
  Yaw_des/1 -> Feedback/3(Yaw_des)
  CornF/1 -> Feedfoward/2(CornF)
  Sum/1 -> Signal Conversion/1
  Feedfoward/1(Mz_FF) -> Gain/1
  Limite min/1 -> Saturation Dynamic/3
  Limite máx/1 -> Saturation Dynamic/1
  Pedal map/1 -> Limite min/1, Limite máx/1, Feedback/4(Pedal map), Feedfoward/5(Pedal map)
  Saturation Dynamic/1 -> To Workspace/1, Mz_ajustado/1
  Signal Conversion/1 -> Saturation Dynamic/2, Scope/1
  Gain/1 -> Sum/2

== system Control_Jetson_10ms_21b 1/Controle/Direct Yaw Control/ON//OFF ==
  Volante : Inport
  TV_On : Inport  Port=2
  Mz_ajustado : Inport  Port=3
  Vx : Inport  Port=4
  Abs : Abs
  Display : Display
  Display1 : Display
  If : If  NumInputs=5  IfExpression=u1<0.05 | u2<1 | u3<2 | u4>0
  If Action Subsystem : Subsystem  TreatAsAtomicUnit=on
  If Action Subsystem1 : Subsystem  TreatAsAtomicUnit=on
  Merge : Merge
  Mz : Outport
  wires:
  Volante/1 -> Abs/1
  Abs/1 -> Display/1, If/1
  Vx/1 -> If/3, Display1/1
  TV_On/1 -> If/2
  If/1 -> If Action Subsystem/Action
  Mz_ajustado/1 -> If/5, If Action Subsystem1/1(Mz_ajustado), If Action Subsystem/1(Mz_ajustado)
  If/2 -> If Action Subsystem1/Action
  If Action Subsystem/1(Mz_OFF) -> Merge/1
  If Action Subsystem1/1(Mz_ON) -> Merge/2
  Merge/1 -> Mz/1
  [Brake] -> If/4

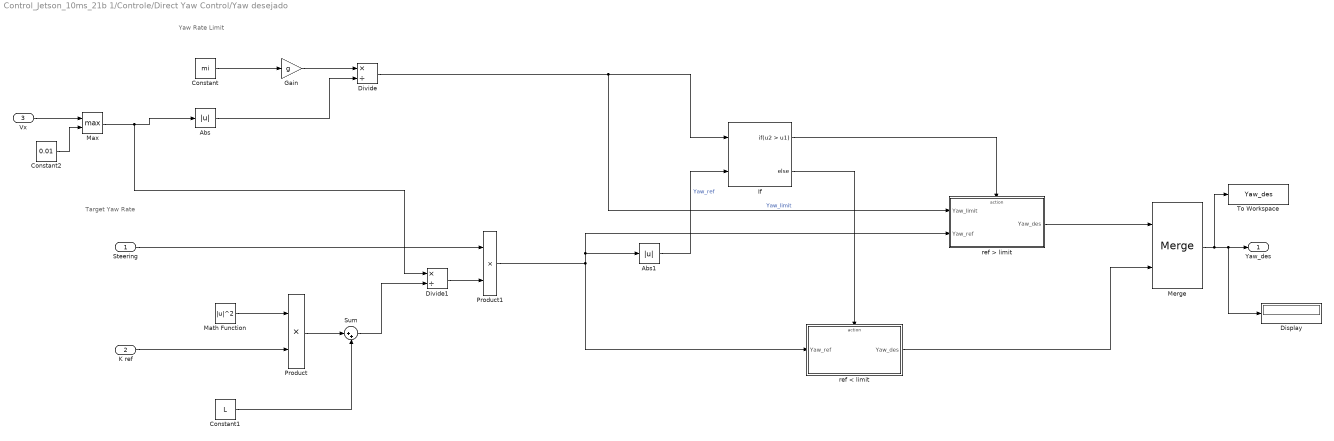
== system Control_Jetson_10ms_21b 1/Controle/Direct Yaw Control/Yaw desejado ==
  note: Target Yaw Rate
  note: Yaw Rate Limit
  Steering : Inport
  K ref : Inport  Port=2
  Vx : Inport  Port=3
  Abs : Abs
  Abs1 : Abs
  Constant : Constant  Value=mi
  Constant1 : Constant  Value=L
  Constant2 : Constant  Value=0.01
  Display : Display
  Divide : Product  Inputs=*/
  Divide1 : Product  Inputs=*/
  Gain : Gain  Gain=g
  If : If  NumInputs=2  IfExpression=u2 > u1
  Math Function : Math  Operator=magnitude^2  SaturateOnIntegerOverflow=on
  Max : MinMax  Function=max  Inputs=2
  Merge : Merge
  Product : Product
  Product1 : Product
  Sum : Sum  Inputs=|++
  To Workspace : ToWorkspace  VariableName=Yaw_des  SaveFormat=Structure With Time  SampleTime=-1
  ref < limit : Subsystem  TreatAsAtomicUnit=on
  ref > limit : Subsystem  TreatAsAtomicUnit=on
  Yaw_des : Outport
  wires:
  Gain/1 -> Divide/1
  Constant/1 -> Gain/1
  Abs/1 -> Divide/2
  Math Function/1 -> Product/1
  K ref/1 -> Product/2
  Product/1 -> Sum/1
  Constant1/1 -> Sum/2
  Sum/1 -> Divide1/2
  Divide1/1 -> Product1/2
  Steering/1 -> Product1/1
  Product1/1 -> ref > limit/2(Yaw_ref), Abs1/1, ref < limit/1(Yaw_ref)
  Divide/1 -> ref > limit/1(Yaw_limit), If/1  "Yaw_limit"
  Abs1/1 -> If/2  "Yaw_ref"
  If/2 -> ref < limit/Action
  If/1 -> ref > limit/Action
  ref < limit/1(Yaw_des) -> Merge/2
  ref > limit/1(Yaw_des) -> Merge/1
  Merge/1 -> To Workspace/1, Display/1, Yaw_des/1
  Vx/1 -> Max/1
  Constant2/1 -> Max/2
  Max/1 -> Divide1/1, Abs/1

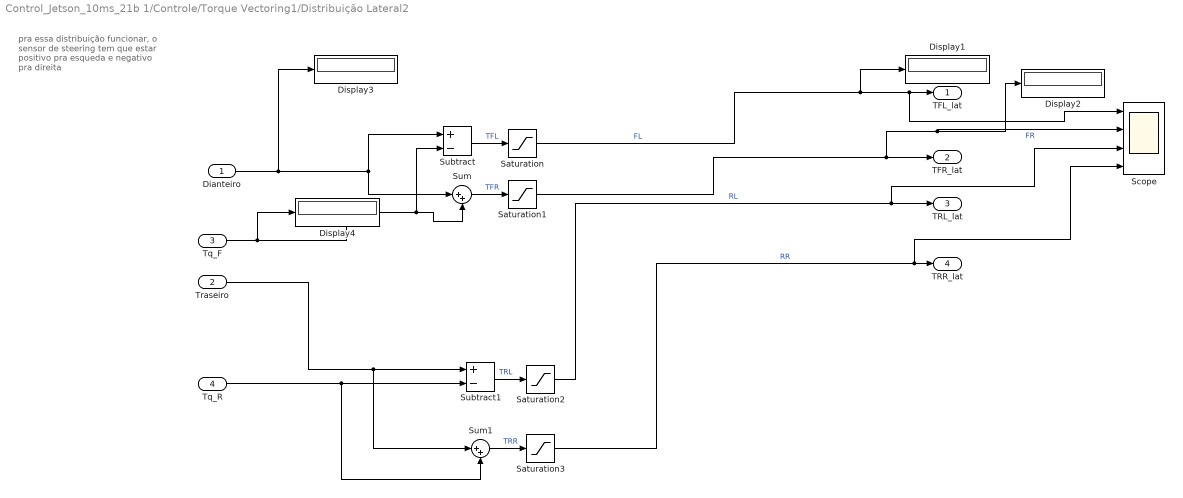
== system Control_Jetson_10ms_21b 1/Controle/Torque Vectoring1/Distribuição Lateral2 ==
  note: pra essa distribuição funcionar, o sensor de steering tem que estar positivo pra esqueda e negativo pra direita
  Dianteiro : Inport
  Traseiro : Inport  Port=2
  Tq_F : Inport  Port=3
  "Tq_R " : Inport  Port=4
  Display{1..4} (4 alike) : Display
  Saturation{,1..3} (4 alike) : Saturate  UpperLimit=14.75  LowerLimit=0
  Scope : Scope  NumInputPorts=4
  Subtract : Sum  Inputs=+-
  Subtract1 : Sum  Inputs=+-
  Sum : Sum  Inputs=|++
  Sum1 : Sum  Inputs=|++
  TFL_lat : Outport
  TFR_lat : Outport  Port=2
  TRL_lat : Outport  Port=3
  TRR_lat : Outport  Port=4
  wires:
  Subtract/1 -> Saturation/1  "TFL"
  "Tq_R "/1 -> Sum1/2, Subtract1/2
  Tq_F/1 -> Display4/1, Sum/2, Subtract/2
  Sum/1 -> Saturation1/1  "TFR"
  Traseiro/1 -> Sum1/1, Subtract1/1
  Sum1/1 -> Saturation3/1  "TRR"
  Subtract1/1 -> Saturation2/1  "TRL"
  Saturation2/1 -> Scope/3, TRL_lat/1  "RL"
  Saturation3/1 -> Scope/4, TRR_lat/1  "RR"
  Dianteiro/1 -> Display3/1, Sum/1, Subtract/1
  Saturation/1 -> Display1/1, Scope/1, TFL_lat/1  "FL"
  Saturation1/1 -> Scope/2, Display2/1, TFR_lat/1  "FR"

== system Control_Jetson_10ms_21b 1/Controle/Torque Vectoring1/Distribuição longitudinal ==
  In1 : Inport
  Constant : Constant
  Display : Display
  Divide : Product  Inputs=*/
  Gain : Gain  Gain=0.25
  Product : Product
  Product1 : Product
  Sum24 : Sum  Inputs=|++
  Sum25 : Sum  Inputs=|++
  Sum26 : Sum  Inputs=+|+
  Dianteiro : Outport
  Traseiro : Outport  Port=2
  tag scope: Theta=global
  wires:
  Sum24/1 -> Sum26/1, Divide/1
  Divide/1 -> [Theta]
  Sum25/1 -> Sum26/2
  Sum26/1 -> Divide/2
  [Fz_FL] -> Sum24/1
  [Fz_RR] -> Sum25/2
  [Fz_FR] -> Sum24/2
  [Fz_RL] -> Sum25/1
  Product1/1 -> Traseiro/1
  Product/1 -> Dianteiro/1
  In1/1 -> Gain/1
  Gain/1 -> Product1/1, Product/2
  Constant/1 -> Product/1, Product1/2

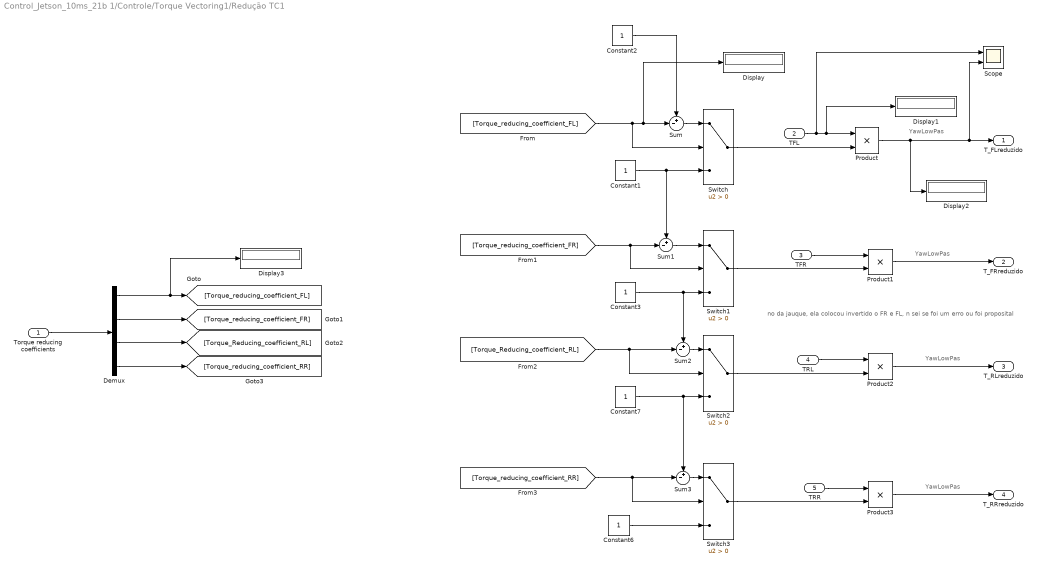
== system Control_Jetson_10ms_21b 1/Controle/Torque Vectoring1/Redução TC1 ==
  note: YawLowPas
  note: no da jauque, ela colocou invertido o FR e FL, n sei se foi um erro ou foi proposital
  note: YawLowPas
  note: YawLowPas
  note: YawLowPas
  Torque reducing coefficients : Inport
  TFL : Inport  Port=2
  TFR : Inport  Port=3
  TRL : Inport  Port=4
  TRR : Inport  Port=5
  Constant{1..3,6..7} (5 alike) : Constant
  Demux : Demux
  Display{,1..3} (4 alike) : Display
  Product{,1..3} (4 alike) : Product
  Scope : Scope  NumInputPorts=2
  Sum{,1..3} (4 alike) : Sum  Inputs=+-|
  Switch{,1..3} (4 alike) : Switch  Criteria=u2 > Threshold
  T_FLreduzido : Outport
  T_FRreduzido : Outport  Port=2
  T_RLreduzido : Outport  Port=3
  T_RRreduzido : Outport  Port=4
  wires:
  Torque reducing coefficients/1 -> Demux/1
  Demux/1 -> Display3/1, [Torque_reducing_coefficient_FL]
  Demux/2 -> [Torque_reducing_coefficient_FR]
  Demux/3 -> [Torque_Reducing_coefficient_RL]
  Demux/4 -> [Torque_reducing_coefficient_RR]
  [Torque_reducing_coefficient_FL] -> Switch/2, Sum/2, Display/1
  Constant1/1 -> Sum1/1, Switch/3
  Switch/1 -> Product/2
  [Torque_reducing_coefficient_FR] -> Sum1/2, Switch1/2
  Constant3/1 -> Switch1/3, Sum2/1
  [Torque_reducing_coefficient_RR] -> Sum3/2, Switch3/2
  [Torque_Reducing_coefficient_RL] -> Sum2/2, Switch2/2
  Constant7/1 -> Sum3/1, Switch2/3
  Constant6/1 -> Switch3/3
  Switch1/1 -> Product1/2
  TFR/1 -> Product1/1
  Switch2/1 -> Product2/2
  TRL/1 -> Product2/1
  Switch3/1 -> Product3/2
  TRR/1 -> Product3/1
  Product1/1 -> T_FRreduzido/1
  Product/1 -> Display2/1, Scope/2, T_FLreduzido/1
  Product2/1 -> T_RLreduzido/1
  Product3/1 -> T_RRreduzido/1
  TFL/1 -> Scope/1, Display1/1, Product/1
  Sum3/1 -> Switch3/1
  Sum2/1 -> Switch2/1
  Sum/1 -> Switch/1
  Sum1/1 -> Switch1/1
  Constant2/1 -> Sum/1

== system Control_Jetson_10ms_21b 1/Controle/Torque Vectoring1/Subsystem ==
  MzT : Inport
  Constant : Constant  Value=Re
  Constant1 : Constant  Value=Gr
  Constant2 : Constant  Value=tr
  Divide : Product  Inputs=*/
  Divide1 : Product  Inputs=*/
  Gain : Gain  Gain=2
  Gain1 : Gain  Gain=2
  Gain2 : Gain  Gain=0.5
  Gain3 : Gain  Gain=0.5
  Product : Product
  Product1 : Product
  Product2 : Product
  Scope : Scope
  Scope1 : Scope  NumInputPorts=2
  tf : Constant  Value=tf
  Tq_F : Outport
  "Tq_R " : Outport  Port=2
  wires:
  MzT/1 -> Product/2, Scope/1
  Constant/1 -> Product/1
  tf/1 -> Product1/1
  Constant1/1 -> Product2/1, Product1/2
  Constant2/1 -> Product2/2
  Product/1 -> Divide/1, Divide1/1
  Product1/1 -> Gain/1
  Product2/1 -> Gain1/1
  Divide/1 -> Gain2/1
  Divide1/1 -> Gain3/1
  Gain/1 -> Divide/2
  Gain1/1 -> Divide1/2
  Gain2/1 -> Scope1/1, Tq_F/1
  Gain3/1 -> Scope1/2, "Tq_R "/1

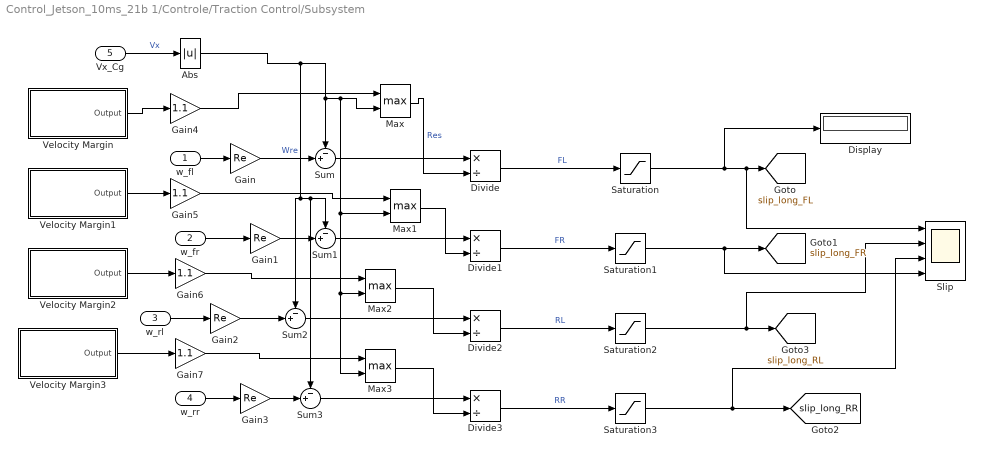
== system Control_Jetson_10ms_21b 1/Controle/Traction Control/Subsystem ==
  w_fl : Inport
  w_fr : Inport  Port=2
  w_rl : Inport  Port=3
  w_rr : Inport  Port=4
  Vx_Cg : Inport  Port=5
  Abs : Abs
  Display : Display
  Divide{,1..3} (4 alike) : Product  Inputs=*/
  Gain{,1..3} (4 alike) : Gain  Gain=Re
  Gain{4..7} (4 alike) : Gain  Gain=1.1
  Max{,1..3} (4 alike) : MinMax  Function=max  Inputs=2
  Saturation{,1..3} (4 alike) : Saturate  UpperLimit=inf  LowerLimit=0
  Slip : Scope  NumInputPorts=4
  Sum{,1..3} (4 alike) : Sum  Inputs=-+|
  Velocity Margin : Subsystem
  Velocity Margin1 : Subsystem
  Velocity Margin2 : Subsystem
  Velocity Margin3 : Subsystem
  tag scope: slip_long_FL=global, slip_long_FR=global, slip_long_RL=global, slip_long_RR=global
  wires:
  Gain7/1 -> Max3/1
  Saturation1/1 -> Slip/4, [slip_long_FR]
  Divide1/1 -> Saturation1/1  "FR"
  Divide/1 -> Saturation/1  "FL"
  Divide3/1 -> Saturation3/1  "RR"
  Velocity Margin3/1(Output) -> Gain7/1
  Gain1/1 -> Sum1/2
  Sum2/1 -> Divide2/1
  Sum/1 -> Divide/1
  Saturation/1 -> Display/1, Slip/1, [slip_long_FL]
  w_rl/1 -> Gain2/1
  Gain6/1 -> Max2/1
  Gain4/1 -> Max/1
  w_fl/1 -> Gain/1
  Sum3/1 -> Divide3/1
  w_fr/1 -> Gain1/1
  Gain5/1 -> Max1/1
  Gain/1 -> Sum/2  "Wre"
  Max2/1 -> Divide2/2
  Vx_Cg/1 -> Abs/1  "Vx"
  Velocity Margin1/1(Output) -> Gain5/1
  Sum1/1 -> Divide1/1
  Gain2/1 -> Sum2/2
  Abs/1 -> Sum3/1, Sum1/1, Sum2/1, Sum/1, Max3/2, Max2/2, Max1/2, Max/2
  Saturation3/1 -> [slip_long_RR], Slip/3
  Velocity Margin/1(Output) -> Gain4/1
  Divide2/1 -> Saturation2/1  "RL"
  Velocity Margin2/1(Output) -> Gain6/1
  Max3/1 -> Divide3/2
  Gain3/1 -> Sum3/2
  w_rr/1 -> Gain3/1
  Max1/1 -> Divide1/2
  Saturation2/1 -> [slip_long_RL], Slip/2
  Max/1 -> Divide/2  "Res"

== system Control_Jetson_10ms_21b 1/Controle/Traction Control/TC_FL ==
  wheel slip : Inport
  Fuzzy Controller : Subsystem
  Rate Limiter : RateLimiter  RisingSlewLimit=inf  SampleTimeMode=inherited
  Torque reducing coefficient : Outport
  wires:
  wheel slip/1 -> Fuzzy Controller/1(wheel slip)
  Fuzzy Controller/1(Torque reducing coefficient) -> Rate Limiter/1
  Rate Limiter/1 -> Torque reducing coefficient/1

== system Control_Jetson_10ms_21b 1/Controle/Traction Control/TC_FR ==
  wheel slip : Inport
  Fuzzy Controller1 : Subsystem
  Rate Limiter : RateLimiter  RisingSlewLimit=inf  SampleTimeMode=inherited
  Torque reducing coefficient : Outport
  wires:
  wheel slip/1 -> Fuzzy Controller1/1(wheel slip)
  Fuzzy Controller1/1(Torque reducing coefficient) -> Rate Limiter/1
  Rate Limiter/1 -> Torque reducing coefficient/1

== system Control_Jetson_10ms_21b 1/Controle/Traction Control/TC_RL ==
  wheel slip : Inport
  Fuzzy Controller : Subsystem
  Rate Limiter : RateLimiter  RisingSlewLimit=inf  SampleTimeMode=inherited
  Torque reducing coefficient : Outport
  wires:
  wheel slip/1 -> Fuzzy Controller/1(wheel slip)
  Fuzzy Controller/1(Torque reducing coefficient) -> Rate Limiter/1
  Rate Limiter/1 -> Torque reducing coefficient/1

== system Control_Jetson_10ms_21b 1/Controle/Traction Control/TC_RR ==
  wheel slip : Inport
  Fuzzy Controller : Subsystem
  Rate Limiter : RateLimiter  RisingSlewLimit=inf  SampleTimeMode=inherited
  Torque reducing coefficient : Outport
  wires:
  wheel slip/1 -> Fuzzy Controller/1(wheel slip)
  Fuzzy Controller/1(Torque reducing coefficient) -> Rate Limiter/1
  Rate Limiter/1 -> Torque reducing coefficient/1

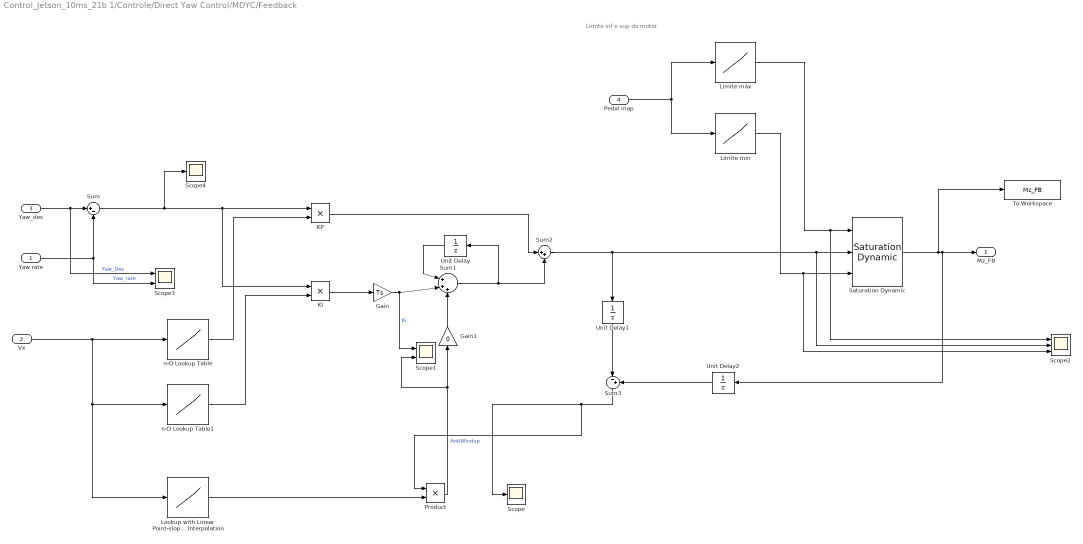
== system Control_Jetson_10ms_21b 1/Controle/Direct Yaw Control/MDYC/Feedback ==
  note: Limite inf e sup do motor
  Yaw rate : Inport
  Vx : Inport  Port=2
  Yaw_des : Inport  Port=3
  Pedal map : Inport  Port=4
  Gain : Gain  Gain=Ts
  Gain1 : Gain  Gain=0
  KI : Product
  KP : Product
  Limite min : Lookup_n-D  NumberOfTableDimensions=1  BreakpointsForDimension1=pedal  BreakpointsForDimension3=[5, 7]  Table=Mz_minF  InternalRulePriority=Speed  RndMeth=Simplest  InputSameDT=on
  Limite máx : Lookup_n-D  NumberOfTableDimensions=1  BreakpointsForDimension1=pedal  BreakpointsForDimension3=[5, 7]  Table=Mz_maxF  InternalRulePriority=Speed  RndMeth=Simplest  InputSameDT=on
  Lookup with Linear Point-slope Interpolation : Lookup_n-D  NumberOfTableDimensions=1  BreakpointsForDimension1=Vx_axis  Table=K_t  InternalRulePriority=Speed  RndMeth=Simplest  InputSameDT=on
  Product : Product
  Saturation Dynamic : simulink/Discontinuities/Saturation Dynamic  OutMin=[]  OutMax=[]  OutDataTypeStr=Inherit: Same as second input  OutDataType=fixdt(1, 16)  OutScaling=2^-10  DoSatur=off
  Scope : Scope
  Scope1 : Scope  NumInputPorts=2
  Scope2 : Scope  NumInputPorts=3
  Scope3 : Scope  NumInputPorts=2
  Scope4 : Scope
  Sum : Sum  Inputs=|+-
  Sum1 : Sum  Inputs=|+++
  Sum2 : Sum  Inputs=|++
  Sum3 : Sum  Inputs=|-+
  To Workspace : ToWorkspace  VariableName=Mz_FB  SaveFormat=Structure With Time  SampleTime=-1
  Unit Delay : UnitDelay  SampleTime=-1  HasFrameUpgradeWarning=on
  Unit Delay1 : UnitDelay  SampleTime=-1  HasFrameUpgradeWarning=on
  Unit Delay2 : UnitDelay  SampleTime=-1  HasFrameUpgradeWarning=on
  n-D Lookup Table : Lookup_n-D  NumberOfTableDimensions=1  BreakpointsForDimension1=Vx_axis  BreakpointsForDimension3=[5, 7]  Table=Kp_data  InternalRulePriority=Speed  RndMeth=Simplest  InputSameDT=on
  n-D Lookup Table1 : Lookup_n-D  NumberOfTableDimensions=1  BreakpointsForDimension1=Vx_axis  BreakpointsForDimension3=[5, 7]  Table=Ki_data  InternalRulePriority=Speed  RndMeth=Simplest  InputSameDT=on
  Mz_FB : Outport
  wires:
  Pedal map/1 -> Limite min/1, Limite máx/1
  Limite máx/1 -> Scope2/1, Saturation Dynamic/1
  Limite min/1 -> Scope2/3, Saturation Dynamic/3
  Yaw_des/1 -> Scope3/1, Sum/1  "Yaw_Des"
  Yaw rate/1 -> Sum/2, Scope3/2  "Yaw_rate"
  n-D Lookup Table/1 -> KP/2
  n-D Lookup Table1/1 -> KI/2
  Sum/1 -> Scope4/1, KI/1, KP/1
  KI/1 -> Gain/1
  Gain/1 -> Scope1/1, Sum1/2  "Ki"
  Unit Delay/1 -> Sum1/1
  Product/1 -> Scope1/2, Gain1/1  "AntiWindup"
  Sum1/1 -> Unit Delay/1, Sum2/2
  KP/1 -> Sum2/1
  Sum3/1 -> Product/1, Scope/1
  Vx/1 -> Lookup with Linear Point-slope Interpolation/1, n-D Lookup Table1/1, n-D Lookup Table/1
  Lookup with Linear Point-slope Interpolation/1 -> Product/2
  Sum2/1 -> Unit Delay1/1, Scope2/2, Saturation Dynamic/2
  Saturation Dynamic/1 -> To Workspace/1, Unit Delay2/1, Mz_FB/1
  Unit Delay1/1 -> Sum3/1
  Unit Delay2/1 -> Sum3/2
  Gain1/1 -> Sum1/3

== system Control_Jetson_10ms_21b 1/Controle/Direct Yaw Control/MDYC/Feedfoward ==
  note: pra não deixar o motor fazer menos que 0 Nm e mais que 21 Nm
  note: Limite inf e sup do motor
  CornR : Inport
  CornF : Inport  Port=2
  K delta : Inport  Port=3
  Ay : Inport  Port=4
  Pedal map : Inport  Port=5
  Add : Sum
  Divide : Product  Inputs=*/
  Gain : Gain  Gain=2*L
  Limite min : Lookup_n-D  NumberOfTableDimensions=1  BreakpointsForDimension1=pedal  BreakpointsForDimension3=[5, 7]  Table=Mz_minF  InternalRulePriority=Speed  RndMeth=Simplest  InputSameDT=on
  Limite máx : Lookup_n-D  NumberOfTableDimensions=1  BreakpointsForDimension1=pedal  BreakpointsForDimension3=[5, 7]  Table=Mz_maxF  InternalRulePriority=Speed  RndMeth=Simplest  InputSameDT=on
  Product : Product
  Product1 : Product
  Product2 : Product
  Saturation Dynamic : simulink/Discontinuities/Saturation Dynamic  OutMin=[]  OutMax=[]  OutDataTypeStr=Inherit: Same as second input  OutDataType=fixdt(1, 16)  OutScaling=2^-10  DoSatur=off
  To Workspace : ToWorkspace  VariableName=Mz_FF  SaveFormat=Structure With Time  SampleTime=-1
  Mz_FF : Outport
  wires:
  Limite min/1 -> Saturation Dynamic/3
  Pedal map/1 -> Limite min/1, Limite máx/1
  Limite máx/1 -> Saturation Dynamic/1
  CornR/1 -> Add/1, Product/1
  CornF/1 -> Add/2, Product/2
  Product/1 -> Gain/1
  Gain/1 -> Divide/1
  Add/1 -> Divide/2
  Divide/1 -> Product1/1
  K delta/1 -> Product1/2
  Product1/1 -> Product2/1
  Product2/1 -> Saturation Dynamic/2
  Saturation Dynamic/1 -> To Workspace/1, Mz_FF/1
  Ay/1 -> Product2/2

== system Control_Jetson_10ms_21b 1/Controle/Direct Yaw Control/ON//OFF/If Action Subsystem ==
  Mz_ajustado : Inport
  Action Port : ActionPort  ActionPortLabel=if(u1<0.05 | u2<1 | u3<2 | u4>0)
  Gain : Gain  Gain=0
  Mz_OFF : Outport
  wires:
  Mz_ajustado/1 -> Gain/1
  Gain/1 -> Mz_OFF/1

== system Control_Jetson_10ms_21b 1/Controle/Direct Yaw Control/ON//OFF/If Action Subsystem1 ==
  Mz_ajustado : Inport
  Action Port : ActionPort  ActionPortLabel=else
  Mz_ON : Outport
  wires:
  Mz_ajustado/1 -> Mz_ON/1

== system Control_Jetson_10ms_21b 1/Controle/Direct Yaw Control/Yaw desejado/ref < limit ==
  Yaw_ref : Inport
  Action Port : ActionPort  ActionPortLabel=else
  Yaw_des : Outport
  wires:
  Yaw_ref/1 -> Yaw_des/1

== system Control_Jetson_10ms_21b 1/Controle/Direct Yaw Control/Yaw desejado/ref > limit ==
  Yaw_limit : Inport
  Yaw_ref : Inport  Port=2
  Action Port : ActionPort  ActionPortLabel=if(u2 > u1)
  Product : Product
  Sign : Signum
  Yaw_des : Outport
  wires:
  Yaw_ref/1 -> Sign/1
  Yaw_limit/1 -> Product/1
  Sign/1 -> Product/2
  Product/1 -> Yaw_des/1

== system Control_Jetson_10ms_21b 1/Controle/Traction Control/Subsystem/Velocity Margin ==
  note: Margin Constant time
  Constant : Constant  Value=Ts
  Gain : Gain  Gain=0.5
  Gain1 : Gain  Gain=(R^2/Iw_+1/M)
  Kx : Subsystem
  Product : Product
  Scope : Scope  NumInputPorts=2
  dfz : Subsystem
  Output : Outport
  wires:
  Constant/1 -> Gain/1
  Gain1/1 -> Product/2
  Product/1 -> Scope/1, Output/1
  [Kx_fl] -> Scope/2, Gain1/1
  Gain/1 -> Product/1

== system Control_Jetson_10ms_21b 1/Controle/Traction Control/Subsystem/Velocity Margin1 ==
  note: Margin Constant time
  Constant : Constant  Value=Ts
  Gain : Gain  Gain=0.5
  Gain1 : Gain  Gain=(R^2/Iw_+1/M)
  Kx : Subsystem
  Product : Product
  dfz : Subsystem
  Output : Outport
  wires:
  Product/1 -> Output/1
  Gain1/1 -> Product/2
  [Kx_fr] -> Gain1/1
  Constant/1 -> Gain/1
  Gain/1 -> Product/1

== system Control_Jetson_10ms_21b 1/Controle/Traction Control/Subsystem/Velocity Margin2 ==
  note: Margin Constant time
  Constant : Constant  Value=Ts
  Gain : Gain  Gain=0.5
  Gain1 : Gain  Gain=(R^2/Iw_+1/M)
  Kx : Subsystem
  Product : Product
  dfz : Subsystem
  Output : Outport
  wires:
  Constant/1 -> Gain/1
  [Kx_rl] -> Gain1/1
  Gain1/1 -> Product/2
  Product/1 -> Output/1
  Gain/1 -> Product/1

== system Control_Jetson_10ms_21b 1/Controle/Traction Control/Subsystem/Velocity Margin3 ==
  note: Margin Constant time
  Constant : Constant  Value=Ts
  Gain : Gain  Gain=0.5
  Gain1 : Gain  Gain=(R^2/Iw_+1/M)
  Kx : Subsystem
  Product : Product
  dfz : Subsystem
  Output : Outport
  wires:
  Product/1 -> Output/1
  Gain1/1 -> Product/2
  Constant/1 -> Gain/1
  [Kx_rr] -> Gain1/1
  Gain/1 -> Product/1

== system Control_Jetson_10ms_21b 1/Controle/Traction Control/TC_FL/Fuzzy Controller ==
  wheel slip : Inport
  Discrete Derivative : simulink/Discrete/Discrete Derivative  gainval=1.0  ICPrevScaledInput=0.0  OutMin=[]  OutMax=[]  OutDataType=fixdt(1, 16)  OutScaling=2^-10  DoSatur=off
  Fuzzy Logic Controller : fuzblock/Fuzzy Logic  Controller  FIS='tc6.fis'  OutputSampleNumber=101  DataType=double  FuzzifiedInputs=off  RuleFiringStrengths=off  RuleOutputs=off  AggregatedOutputs=off  SimulateUsing=Code generation  OutOfRangeInputValueMessage=warning  NoRuleFiredMessage=warning  EmptyOutputFuzzySetMessage=warning
  Mux1 : Mux  Inputs=2
  Saturation : Saturate  UpperLimit=1  LowerLimit=0
  Scope : Scope
  Scope1 : Scope
  Scope2 : Scope  NumInputPorts=2
  Torque reducing coefficient : Outport
  wires:
  Mux1/1 -> Fuzzy Logic Controller/1
  Fuzzy Logic Controller/1 -> Saturation/1, Scope2/1
  Saturation/1 -> Scope2/2, Torque reducing coefficient/1
  Discrete Derivative/1 -> Scope1/1, Mux1/2
  wheel slip/1 -> Scope/1, Mux1/1, Discrete Derivative/1

== system Control_Jetson_10ms_21b 1/Controle/Traction Control/TC_FR/Fuzzy Controller1 ==
  wheel slip : Inport
  Discrete Derivative : simulink/Discrete/Discrete Derivative  Commented=on  gainval=1.0  ICPrevScaledInput=0.0  OutMin=[]  OutMax=[]  OutDataType=fixdt(1, 16)  OutScaling=2^-10  DoSatur=off
  Discrete Derivative1 : simulink/Discrete/Discrete Derivative  gainval=1.0  ICPrevScaledInput=0.0  OutMin=[]  OutMax=[]  OutDataType=fixdt(1, 16)  OutScaling=2^-10  DoSatur=off
  Fuzzy Logic Controller : fuzblock/Fuzzy Logic  Controller  FIS='tc6.fis'  OutputSampleNumber=101  DataType=double  FuzzifiedInputs=off  RuleFiringStrengths=off  RuleOutputs=off  AggregatedOutputs=off  SimulateUsing=Code generation  OutOfRangeInputValueMessage=warning  NoRuleFiredMessage=warning  EmptyOutputFuzzySetMessage=warning
  Mux1 : Mux  Inputs=2
  Saturation : Saturate  UpperLimit=1  LowerLimit=0
  Scope : Scope  NumInputPorts=3
  Torque reducing coefficient : Outport
  wires:
  Mux1/1 -> Fuzzy Logic Controller/1
  Fuzzy Logic Controller/1 -> Saturation/1, Scope/3  "red"
  Discrete Derivative1/1 -> Mux1/2, Scope/2  "der"
  wheel slip/1 -> Mux1/1, Scope/1, Discrete Derivative1/1  "slip"
  Saturation/1 -> Torque reducing coefficient/1

== system Control_Jetson_10ms_21b 1/Controle/Traction Control/TC_RL/Fuzzy Controller ==
  wheel slip : Inport
  Discrete Derivative : simulink/Discrete/Discrete Derivative  Commented=on  gainval=1.0  ICPrevScaledInput=0.0  OutMin=[]  OutMax=[]  OutDataType=fixdt(1, 16)  OutScaling=2^-10  DoSatur=off
  Discrete Derivative1 : simulink/Discrete/Discrete Derivative  gainval=1.0  ICPrevScaledInput=0.0  OutMin=[]  OutMax=[]  OutDataType=fixdt(1, 16)  OutScaling=2^-10  DoSatur=off
  Fuzzy Logic Controller : fuzblock/Fuzzy Logic  Controller  FIS='tc6.fis'  OutputSampleNumber=101  DataType=double  FuzzifiedInputs=off  RuleFiringStrengths=off  RuleOutputs=off  AggregatedOutputs=off  SimulateUsing=Code generation  OutOfRangeInputValueMessage=warning  NoRuleFiredMessage=warning  EmptyOutputFuzzySetMessage=warning
  Mux : Mux  Inputs=2
  Saturation : Saturate  UpperLimit=1  LowerLimit=0
  Scope : Scope  NumInputPorts=3
  Torque reducing coefficient : Outport
  wires:
  Mux/1 -> Fuzzy Logic Controller/1
  Fuzzy Logic Controller/1 -> Saturation/1, Scope/3
  Saturation/1 -> Torque reducing coefficient/1
  Discrete Derivative1/1 -> Mux/2, Scope/2
  wheel slip/1 -> Scope/1, Mux/1, Discrete Derivative1/1

== system Control_Jetson_10ms_21b 1/Controle/Traction Control/TC_RR/Fuzzy Controller ==
  wheel slip : Inport
  Discrete Derivative : simulink/Discrete/Discrete Derivative  Commented=on  gainval=1.0  ICPrevScaledInput=0.0  OutMin=[]  OutMax=[]  OutDataType=fixdt(1, 16)  OutScaling=2^-10  DoSatur=off
  Discrete Derivative1 : simulink/Discrete/Discrete Derivative  gainval=1.0  ICPrevScaledInput=0.0  OutMin=[]  OutMax=[]  OutDataType=fixdt(1, 16)  OutScaling=2^-10  DoSatur=off
  Fuzzy Logic Controller1 : fuzblock/Fuzzy Logic  Controller  FIS='tc6.fis'  OutputSampleNumber=101  DataType=double  FuzzifiedInputs=off  RuleFiringStrengths=off  RuleOutputs=off  AggregatedOutputs=off  SimulateUsing=Code generation  OutOfRangeInputValueMessage=warning  NoRuleFiredMessage=warning  EmptyOutputFuzzySetMessage=warning
  Mux : Mux  Inputs=2
  Saturation : Saturate  UpperLimit=1  LowerLimit=0
  Scope : Scope  NumInputPorts=3
  Torque reducing coefficient : Outport
  wires:
  Mux/1 -> Fuzzy Logic Controller1/1
  Fuzzy Logic Controller1/1 -> Saturation/1, Scope/3
  Saturation/1 -> Torque reducing coefficient/1
  Discrete Derivative1/1 -> Mux/2, Scope/2
  wheel slip/1 -> Mux/1, Scope/1, Discrete Derivative1/1

== system Control_Jetson_10ms_21b 1/Controle/Traction Control/Subsystem/Velocity Margin/Kx ==
  Constant : Constant  Value=kx1  SampleTime=0.01
  Exp : Math  SaturateOnIntegerOverflow=on
  Gain : Gain  Gain=kx3
  Gain1 : Gain  Gain=kx2
  Gain2 : Gain  Gain=-1
  Gain3 : Gain  Gain=1+px3*dpi+px4*dpi^2
  Product : Product
  Product1 : Product
  Scope : Scope
  Scope1 : Scope
  Scope2 : Scope
  Sum : Sum  Inputs=|++
  tag scope: Kx_fl=global
  wires:
  [Fz_FL] -> Gain2/1
  Product/1 -> Product1/1
  Exp/1 -> Scope/1, Product1/2
  Gain1/1 -> Sum/2
  Sum/1 -> Scope2/1, Product/2
  Product1/1 -> Gain3/1
  Constant/1 -> Sum/1
  Gain/1 -> Exp/1
  [dfz_fl] -> Gain1/1, Gain/1
  Gain2/1 -> Product/1
  Gain3/1 -> Scope1/1, [Kx_fl]

== system Control_Jetson_10ms_21b 1/Controle/Traction Control/Subsystem/Velocity Margin/dfz ==
  Constant : Constant  Value=Fz0x
  Display : Display
  Display1 : Display
  Divide : Product  Inputs=*/
  Gain : Gain  Gain=-1
  Scope : Scope  NumInputPorts=2
  Sum : Sum  Inputs=|+-
  tag scope: dfz_fl=global
  wires:
  Constant/1 -> Divide/2, Sum/2
  Sum/1 -> Divide/1
  Divide/1 -> Display1/1, Scope/2, [dfz_fl]
  [Fz_FL] -> Gain/1
  Gain/1 -> Scope/1, Display/1, Sum/1

== system Control_Jetson_10ms_21b 1/Controle/Traction Control/Subsystem/Velocity Margin1/Kx ==
  Constant : Constant  Value=kx1
  Exp : Math  SaturateOnIntegerOverflow=on
  Gain : Gain  Gain=kx3
  Gain1 : Gain  Gain=kx2
  Gain2 : Gain  Gain=-1
  Gain3 : Gain  Gain=1+px3*dpi+px4*dpi^2
  Product : Product
  Product1 : Product
  Sum : Sum  Inputs=|++
  tag scope: Kx_fr=global
  wires:
  Constant/1 -> Sum/1
  Product1/1 -> Gain3/1
  Sum/1 -> Product/2
  Gain1/1 -> Sum/2
  Exp/1 -> Product1/2
  Product/1 -> Product1/1
  [Fz_FR] -> Gain2/1
  Gain/1 -> Exp/1
  [dfz_fr] -> Gain1/1, Gain/1
  Gain2/1 -> Product/1
  Gain3/1 -> [Kx_fr]

== system Control_Jetson_10ms_21b 1/Controle/Traction Control/Subsystem/Velocity Margin1/dfz ==
  Constant : Constant  Value=Fz0x
  Divide : Product  Inputs=*/
  Gain : Gain  Gain=-1
  Sum : Sum  Inputs=|+-
  tag scope: dfz_fr=global
  wires:
  Divide/1 -> [dfz_fr]
  Sum/1 -> Divide/1
  Constant/1 -> Sum/2, Divide/2
  [Fz_FR] -> Gain/1
  Gain/1 -> Sum/1

== system Control_Jetson_10ms_21b 1/Controle/Traction Control/Subsystem/Velocity Margin2/Kx ==
  Constant : Constant  Value=kx1
  Exp : Math  SaturateOnIntegerOverflow=on
  Gain : Gain  Gain=kx3
  Gain1 : Gain  Gain=kx2
  Gain2 : Gain  Gain=-1
  Gain3 : Gain  Gain=1+px3*dpi+px4*dpi^2
  Product : Product
  Product1 : Product
  Sum : Sum  Inputs=|++
  tag scope: Kx_rl=global
  wires:
  Constant/1 -> Sum/1
  Product1/1 -> Gain3/1
  Sum/1 -> Product/2
  Gain1/1 -> Sum/2
  Exp/1 -> Product1/2
  Product/1 -> Product1/1
  [Fz_RL] -> Gain2/1
  Gain/1 -> Exp/1
  [dfz_rl] -> Gain1/1, Gain/1
  Gain2/1 -> Product/1
  Gain3/1 -> [Kx_rl]

== system Control_Jetson_10ms_21b 1/Controle/Traction Control/Subsystem/Velocity Margin2/dfz ==
  Constant : Constant  Value=Fz0x
  Divide : Product  Inputs=*/
  Gain : Gain  Gain=-1
  Sum : Sum  Inputs=|+-
  tag scope: dfz_rl=global
  wires:
  Divide/1 -> [dfz_rl]
  Sum/1 -> Divide/1
  Constant/1 -> Sum/2, Divide/2
  [Fz_RL] -> Gain/1
  Gain/1 -> Sum/1

== system Control_Jetson_10ms_21b 1/Controle/Traction Control/Subsystem/Velocity Margin3/Kx ==
  Constant : Constant  Value=kx1
  Exp : Math  SaturateOnIntegerOverflow=on
  Gain : Gain  Gain=kx3
  Gain1 : Gain  Gain=kx2
  Gain2 : Gain  Gain=-1
  Gain3 : Gain  Gain=1+px3*dpi+px4*dpi^2
  Product : Product
  Product1 : Product
  Sum : Sum  Inputs=|++
  tag scope: Kx_rr=global
  wires:
  [Fz_RR] -> Gain2/1
  Product/1 -> Product1/1
  Exp/1 -> Product1/2
  Gain1/1 -> Sum/2
  Sum/1 -> Product/2
  Product1/1 -> Gain3/1
  Constant/1 -> Sum/1
  Gain/1 -> Exp/1
  [dfz_rr] -> Gain1/1, Gain/1
  Gain2/1 -> Product/1
  Gain3/1 -> [Kx_rr]
